simulink model "stereo_ibvs_sim_stage1"  (R2025b)
settings: Solver=FixedStepDiscrete  StartTime=0  StopTime=6  FixedStep=cfg.Ts  RelTol=1e-3
InitFcn:
  | addpath('/home/harry/franka_ros2_ws/src/visual_servo_tag/simulink/core');addpath('/home/harry/franka_ros2_ws/src/visual_servo_tag/simulink/config');assignin('base','STEREO_IBVS_SIMULATION_MODE',true);run('/home/harry/franka_ros2_ws/src/visual_servo_tag/simulink/config/stereo_ibvs_config.m');
StopFcn:
  | assignin('base','STEREO_IBVS_SIMULATION_MODE',false);run('/home/harry/franka_ros2_ws/src/visual_servo_tag/simulink/config/stereo_ibvs_config.m');
values from neighbouring files (symbols this model uses):
  cfg = evalin('base','cfg')    [plot_stereo_ibvs_sim_stage1_results.m]
CloseFcn:
  | assignin('base','STEREO_IBVS_SIMULATION_MODE',false);run('/home/harry/franka_ros2_ws/src/visual_servo_tag/simulink/config/stereo_ibvs_config.m');
settings Model: Creator=harry  LastModifiedBy=harry

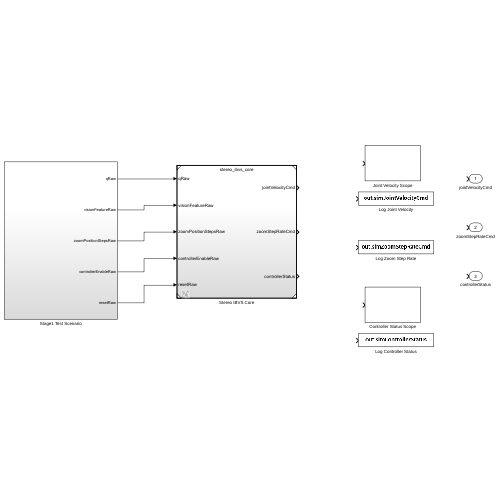
[thumbnail: Simulink's stored preview of the top-level diagram]
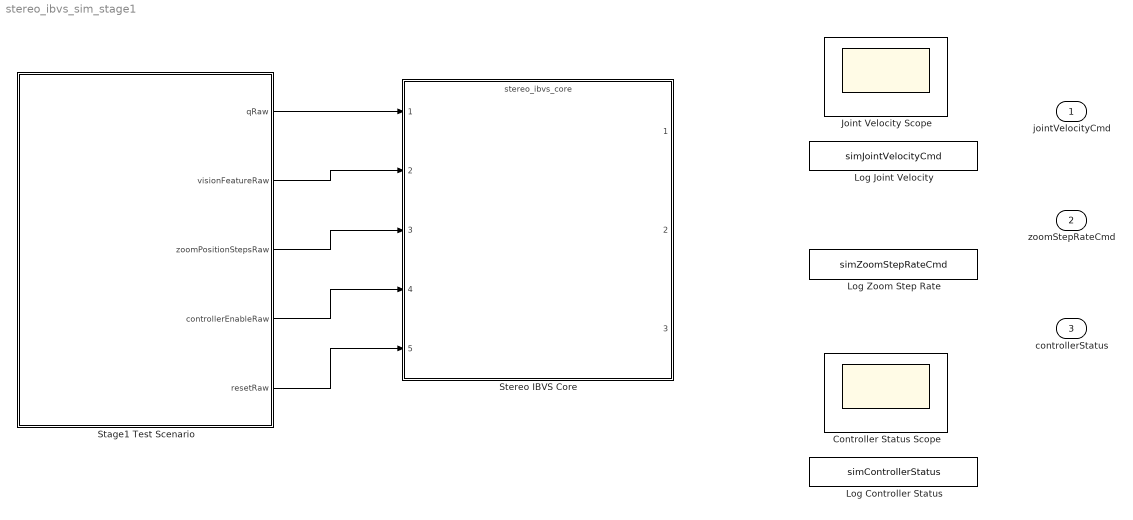
== system stereo_ibvs_sim_stage1 ==
  Controller Status Scope : Scope
  Joint Velocity Scope : Scope
  Log Controller Status : ToWorkspace  VariableName=simControllerStatus  SaveFormat=Timeseries  SampleTime=-1
  Log Joint Velocity : ToWorkspace  VariableName=simJointVelocityCmd  SaveFormat=Timeseries  SampleTime=-1
  Log Zoom Step Rate : ToWorkspace  VariableName=simZoomStepRateCmd  SaveFormat=Timeseries  SampleTime=-1
  Stage1 Test Scenario : Subsystem
  Stereo IBVS Core : ModelReference  ModelNameDialog=stereo_ibvs_core  SimulationMode=Normal  ModelReferenceVersion=1.47
  jointVelocityCmd : Outport  PortDimensions=[7 1]
  zoomStepRateCmd : Outport  Port=2  PortDimensions=[2 1]
  controllerStatus : Outport  Port=3  PortDimensions=[12 1]
  wires:
  Stage1 Test Scenario/1(qRaw) -> Stereo IBVS Core/1
  Stage1 Test Scenario/2(visionFeatureRaw) -> Stereo IBVS Core/2
  Stage1 Test Scenario/3(zoomPositionStepsRaw) -> Stereo IBVS Core/3
  Stage1 Test Scenario/4(controllerEnableRaw) -> Stereo IBVS Core/4
  Stage1 Test Scenario/5(resetRaw) -> Stereo IBVS Core/5

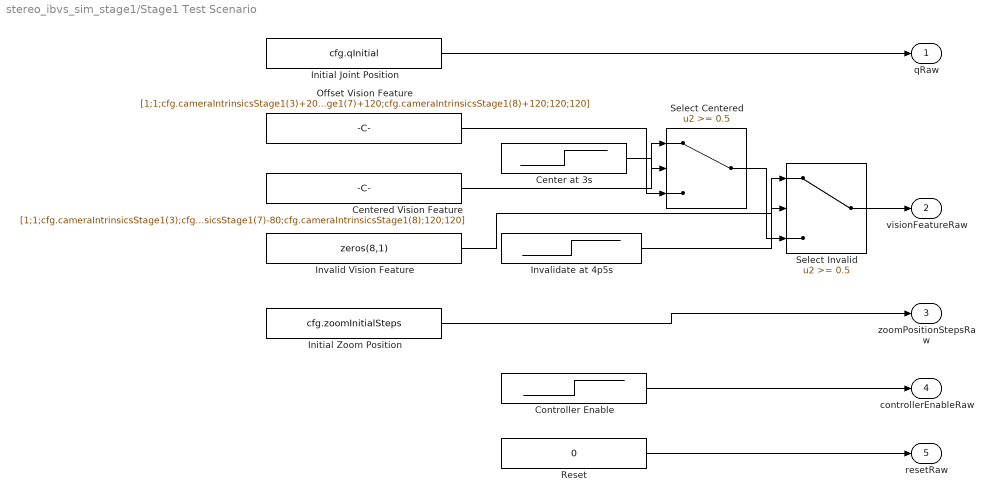
== system stereo_ibvs_sim_stage1/Stage1 Test Scenario ==
  Center at 3s : Step  Time=3  SampleTime=cfg.Ts
  Centered Vision Feature : Constant  Value=[1;1;cfg.cameraIntrinsicsStage1(3);cfg.cameraIntrinsicsStage1(4);cfg.cameraIntrinsicsStage1(7)-80;cfg.cameraIntrinsicsStage1(8);120;120]  VectorParams1D=off  OutDataTypeStr=double  SampleTime=cfg.Ts
  Controller Enable : Step  Time=0.5  SampleTime=cfg.Ts
  Initial Joint Position : Constant  Value=cfg.qInitial  VectorParams1D=off  OutDataTypeStr=double  SampleTime=cfg.Ts
  Initial Zoom Position : Constant  Value=cfg.zoomInitialSteps  VectorParams1D=off  OutDataTypeStr=double  SampleTime=cfg.Ts
  Invalid Vision Feature : Constant  Value=zeros(8,1)  VectorParams1D=off  OutDataTypeStr=double  SampleTime=cfg.Ts
  Invalidate at 4p5s : Step  Time=4.5  SampleTime=cfg.Ts
  Offset Vision Feature : Constant  Value=[1;1;cfg.cameraIntrinsicsStage1(3)+200;cfg.cameraIntrinsicsStage1(4)+120;cfg.cameraIntrinsicsStage1(7)+120;cfg.cameraIntrinsicsStage1(8)+120;120;120]  VectorParams1D=off  OutDataTypeStr=double  SampleTime=cfg.Ts
  Reset : Constant  Value=0  OutDataTypeStr=double  SampleTime=cfg.Ts
  Select Centered : Switch  Threshold=0.5  SaturateOnIntegerOverflow=off  InputSameDT=off
  Select Invalid : Switch  Threshold=0.5  SaturateOnIntegerOverflow=off  InputSameDT=off
  qRaw : Outport  PortDimensions=[7 1]
  visionFeatureRaw : Outport  Port=2  PortDimensions=[8 1]
  zoomPositionStepsRaw : Outport  Port=3  PortDimensions=[2 1]
  controllerEnableRaw : Outport  Port=4  PortDimensions=1
  resetRaw : Outport  Port=5  PortDimensions=1
  wires:
  Centered Vision Feature/1 -> Select Centered/1
  Center at 3s/1 -> Select Centered/2
  Offset Vision Feature/1 -> Select Centered/3
  Invalid Vision Feature/1 -> Select Invalid/1
  Invalidate at 4p5s/1 -> Select Invalid/2
  Select Centered/1 -> Select Invalid/3
  Initial Joint Position/1 -> qRaw/1
  Select Invalid/1 -> visionFeatureRaw/1
  Initial Zoom Position/1 -> zoomPositionStepsRaw/1
  Controller Enable/1 -> controllerEnableRaw/1
  Reset/1 -> resetRaw/1
